simulink model "CommGov"  (R2021a)
settings: Solver=VariableStepDiscrete  StartTime=0.0  StopTime=10  RelTol=1e-3
undefined symbols (not defined in the file): A_ol, B_ol, dt, Gx, Hv, hv, Hx, r, x0
settings Model: Creator=mani8618  LastModifiedBy=mani8618

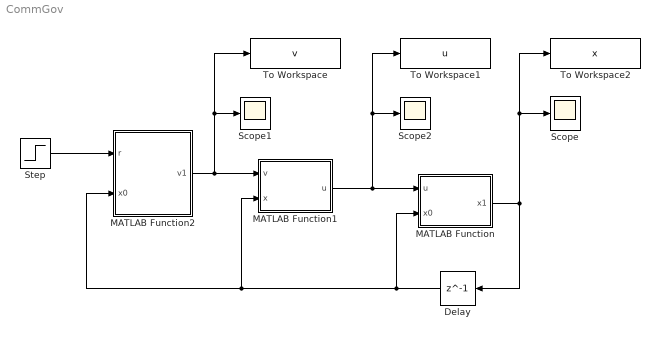
== system CommGov ==
  Delay : Delay  DelayLength=1  InitialCondition=x0  SampleTime=dt
  MATLAB Function : MATLAB Function  TreatAsAtomicUnit=on
  MATLAB Function1 : MATLAB Function  TreatAsAtomicUnit=on
  MATLAB Function2 : MATLAB Function  TreatAsAtomicUnit=on
  Scope : Scope
  Scope1 : Scope
  Scope2 : Scope
  Step : Step  Before=Gx\x0  After=r  SampleTime=0
  To Workspace : ToWorkspace  VariableName=v  SampleTime=-1
  To Workspace1 : ToWorkspace  VariableName=u  SampleTime=-1
  To Workspace2 : ToWorkspace  VariableName=x  SampleTime=-1
  wires:
  MATLAB Function/1(x1) -> To Workspace2/1, Scope/1, Delay/1
  MATLAB Function1/1(u) -> MATLAB Function/1(u), To Workspace1/1, Scope2/1
  Step/1 -> MATLAB Function2/1(r)
  Delay/1 -> MATLAB Function1/2(x), MATLAB Function2/2(x0), MATLAB Function/2(x0)
  MATLAB Function2/1(v1) -> MATLAB Function1/1(v), Scope1/1, To Workspace/1

== matlab function CommGov/MATLAB Function1 ==
  data: v input; x input; u output; K parameter
function u = fcn(v,x,K)

% u = -kp*(x(1)-v)-kd*x(2);

u = -K*[(x(1)-v);x(2)];

end

== matlab function CommGov/MATLAB Function ==
  data: u input; x0 input; x1 output; A_ol parameter; B_ol parameter
function x1 = fcn(u,x0,A_ol, B_ol)

x1 = A_ol*x0+B_ol*u;

end

== matlab function CommGov/MATLAB Function2 ==
  data: r input; x0 input; Hx parameter; v1 output; Hv parameter; hv parameter
function v1 = fcn(r,x0,Hx,Hv,hv)
coder.extrinsic('quadprog')
coder.extrinsic('optimoptions')

v1 = r;
v1 = quadprog(1,-r,Hv,hv-Hx*x0,[],[],[],[],[],optimoptions('quadprog','Display','none'));

end
